simulink model "spoolingControllerVDL"  (R2022a)
settings: Solver=VariableStepAuto  StartTime=0.0  StopTime=10.0  RelTol=1e-3
undefined symbols (not defined in the file or in its folder): desThrLen, wnch
settings Model: Creator=adabney  LastModifiedBy=jbfine

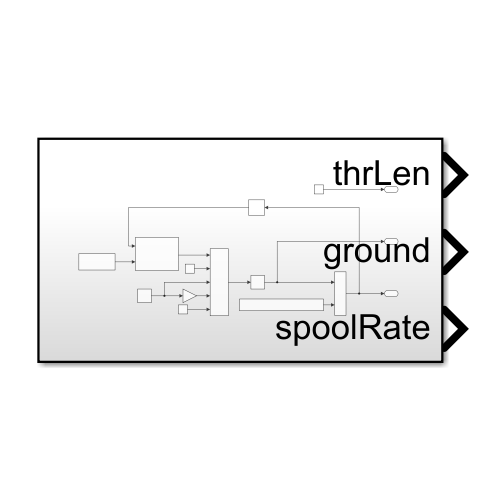
[thumbnail: Simulink's stored preview of the top-level diagram]
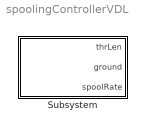
== system spoolingControllerVDL ==
  Subsystem : Subsystem

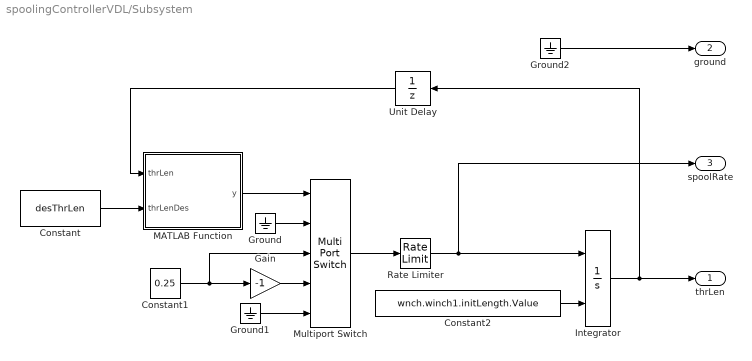
== system spoolingControllerVDL/Subsystem ==
  Constant : Constant  Value=desThrLen
  Constant1 : Constant  Value=0.25
  Constant2 : Constant  Value=wnch.winch1.initLength.Value  VectorParams1D=off
  Gain : Gain  Gain=-1
  Ground : Ground
  Ground1 : Ground
  Ground2 : Ground
  Integrator : Integrator  InitialConditionSource=external
  MATLAB Function : MATLAB Function  TreatAsAtomicUnit=on
  Multiport Switch : MultiPortSwitch  DataPortForDefault=Additional data port  SaturateOnIntegerOverflow=off  InputSameDT=off
  Rate Limiter : RateLimiter  RisingSlewLimit=.125  FallingSlewLimit=-.125  SampleTimeMode=inherited
  Unit Delay : UnitDelay  SampleTime=-1  HasFrameUpgradeWarning=on
  thrLen : Outport
  ground : Outport  Port=2
  spoolRate : Outport  Port=3
  wires:
  Gain/1 -> Multiport Switch/4
  Rate Limiter/1 -> spoolRate/1, Integrator/1
  Constant1/1 -> Multiport Switch/3, Gain/1
  Multiport Switch/1 -> Rate Limiter/1
  Integrator/1 -> thrLen/1, Unit Delay/1
  Constant2/1 -> Integrator/2
  Unit Delay/1 -> MATLAB Function/1(thrLen)
  MATLAB Function/1(y) -> Multiport Switch/1
  Ground/1 -> Multiport Switch/2
  Constant/1 -> MATLAB Function/2(thrLenDes)
  Ground1/1 -> Multiport Switch/5
  Ground2/1 -> ground/1

== matlab function spoolingControllerVDL/Subsystem/MATLAB Function ==
  data: thrLen input; thrLenDes input; y output
function y = fcn(thrLen, thrLenDes)

err = thrLenDes-thrLen;

if abs(err)< 0.1
    y = 1;
elseif err > 0.1
    y = 2;
else
    y = 3;
end
